simulink model "mZoom"  (Simulink 7.1)
settings: Solver=FixedStepDiscrete  StartTime=0.0  StopTime=10.0  FixedStep=0.1  RelTol=1e-3
settings Model: Creator=jcobleig  LastModifiedBy=jcobleig
settings DataIOCC: SaveOutput=off  SignalLogging=off  SaveTime=off
settings OptimizationCC: InlineParams=on
settings DebuggingCC: StrictBusMsg=ErrorOnBusTreatedAsVector

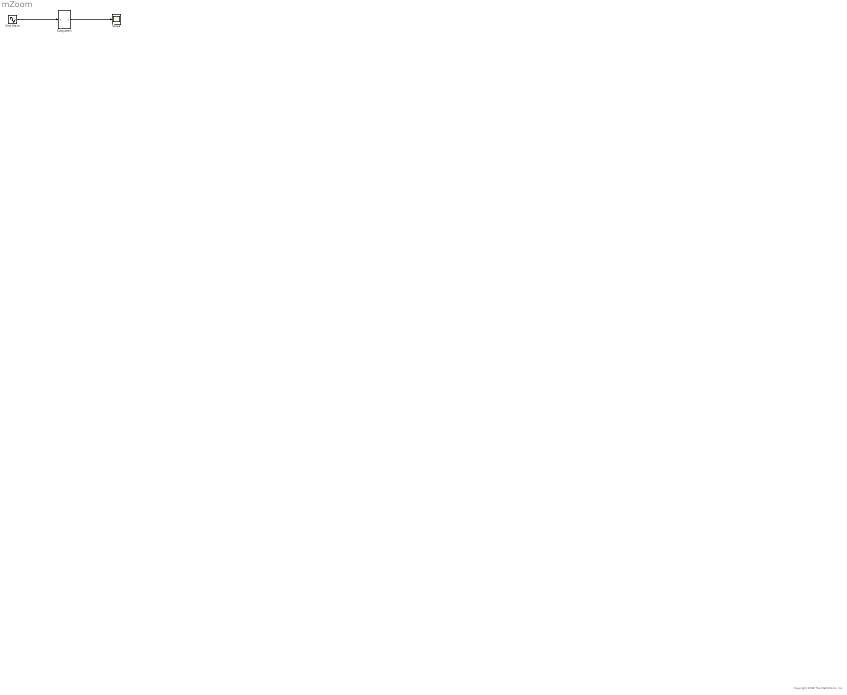
== system mZoom ==
  note: Copyright 2008 The MathWorks, Inc.
  Scope : Scope
  Sine Wave : Sin  SampleTime=0.1
  Subsystem : Subsystem
  wires:
  Sine Wave/1 -> Subsystem/1(In1)
  Subsystem/1(Out1) -> Scope/1

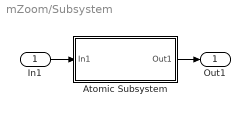
== system mZoom/Subsystem ==
  In1 : Inport
  Atomic Subsystem : Subsystem  TreatAsAtomicUnit=on
  Out1 : Outport
  wires:
  In1/1 -> Atomic Subsystem/1(In1)
  Atomic Subsystem/1(Out1) -> Out1/1

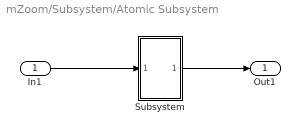
== system mZoom/Subsystem/Atomic Subsystem ==
  In1 : Inport  SampleTime=0.1  OutDataType=sfix(16)  OutScaling=2^0
  Subsystem : Subsystem
  Out1 : Outport  OutDataType=sfix(16)  OutScaling=2^0
  wires:
  In1/1 -> Subsystem/1(In1)
  Subsystem/1(Out1) -> Out1/1

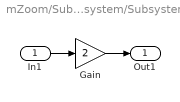
== system mZoom/Subsystem/Atomic Subsystem/Subsystem ==
  In1 : Inport
  Gain : Gain  Gain=2  ParameterDataType=sfix(16)  ParameterScaling=2^0  OutDataType=sfix(16)  OutScaling=2^0
  Out1 : Outport
  wires:
  In1/1 -> Gain/1
  Gain/1 -> Out1/1
